simulink model "z_sim"  (R2018b)
settings: Solver=VariableStepAuto  StartTime=0.0  StopTime=10  RelTol=1e-3
values from neighbouring files (symbols this model uses):
  tau = 0.8419    [lab2.m]    (also in lab2.mat = 0.841912607087)
  z1 = z(i)    [lab2.m]    (also in lab2.mat = -16.6)
  z2 = z1 / 2    [lab2.m]    (also in lab2.mat = -8.3)
  z3 = z1 / 3    [lab2.m]    (also in lab2.mat = -5.53333333333)
settings Model: Creator=EE103  LastModifiedBy=Oguz
settings SFSimCC: SimUseLocalCustomCode=off
settings RTWCC: RTWUseLocalCustomCode=off
settings CodeAppCC: StateflowObjectComments=on

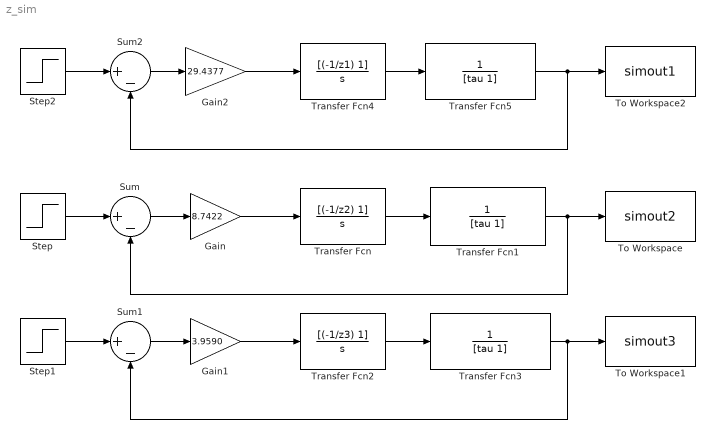
== system z_sim ==
  Gain : Gain  Gain=8.7422
  Gain1 : Gain  Gain=3.9590
  Gain2 : Gain  Gain=29.4377
  Step : Step  Time=0  After=50  SampleTime=0.01
  Step1 : Step  Time=0  After=50  SampleTime=0.01
  Step2 : Step  Time=0  After=50  SampleTime=0.01
  Sum : Sum  Inputs=|+-
  Sum1 : Sum  Inputs=|+-
  Sum2 : Sum  Inputs=|+-
  To Workspace : ToWorkspace  VariableName=simout2  SaveFormat=Timeseries  SampleTime=-1
  To Workspace1 : ToWorkspace  VariableName=simout3  SaveFormat=Timeseries  SampleTime=-1
  To Workspace2 : ToWorkspace  VariableName=simout1  SaveFormat=Timeseries  SampleTime=-1
  Transfer Fcn : TransferFcn  Numerator=[(-1/z2) 1]  Denominator=[1 0]
  Transfer Fcn1 : TransferFcn  Denominator=[tau 1]
  Transfer Fcn2 : TransferFcn  Numerator=[(-1/z3) 1]  Denominator=[1 0]
  Transfer Fcn3 : TransferFcn  Denominator=[tau 1]
  Transfer Fcn4 : TransferFcn  Numerator=[(-1/z1) 1]  Denominator=[1 0]
  Transfer Fcn5 : TransferFcn  Denominator=[tau 1]
  wires:
  Gain/1 -> Transfer Fcn/1
  Transfer Fcn/1 -> Transfer Fcn1/1
  Step/1 -> Sum/1
  Sum/1 -> Gain/1
  Transfer Fcn1/1 -> Sum/2, To Workspace/1
  Gain1/1 -> Transfer Fcn2/1
  Transfer Fcn2/1 -> Transfer Fcn3/1
  Step1/1 -> Sum1/1
  Sum1/1 -> Gain1/1
  Transfer Fcn3/1 -> Sum1/2, To Workspace1/1
  Gain2/1 -> Transfer Fcn4/1
  Transfer Fcn4/1 -> Transfer Fcn5/1
  Step2/1 -> Sum2/1
  Sum2/1 -> Gain2/1
  Transfer Fcn5/1 -> Sum2/2, To Workspace2/1
